simulink model "yoyomodel"  (R2023a)
settings: Solver=VariableStepAuto  StartTime=0.0  StopTime=inf  RelTol=1e-3
values from neighbouring files (symbols this model uses):
  A = [0 ,1; 0, -(e*r)/(I + m*r^2)]    [yoyo.m]
  B = [0; 1/(I + m*r^2)]    [yoyo.m]
  Bi = 1/32.5494    (= 0.0307225325198)    [yoyo.m]
  C = [1 ,0]    [yoyo.m]
  g = 9.81    [yoyo.m]
  K = acker(A,B,[0 0])    [yoyo.m]
  L = acker(A_ccf',C_ccf', [-0.01 -0.01])'    [yoyo.m]
  m = 0.1    [yoyo.m]
  r = 0.035    [yoyo.m]
  x0 = [0; 0]    [yoyo.m]
settings Model: Creator=aditya  LastModifiedBy=aditya
settings SolverCC: ZeroCrossAlgorithm=Adaptive
settings DataIOCC: Refine=5
settings DebuggingCC: IgnoredZcDiagnostic=none

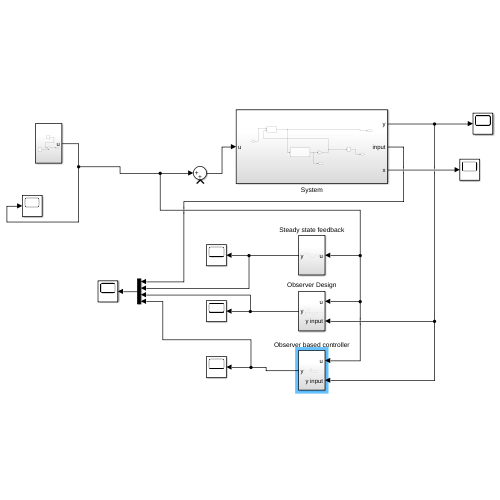
[thumbnail: Simulink's stored preview of the top-level diagram]
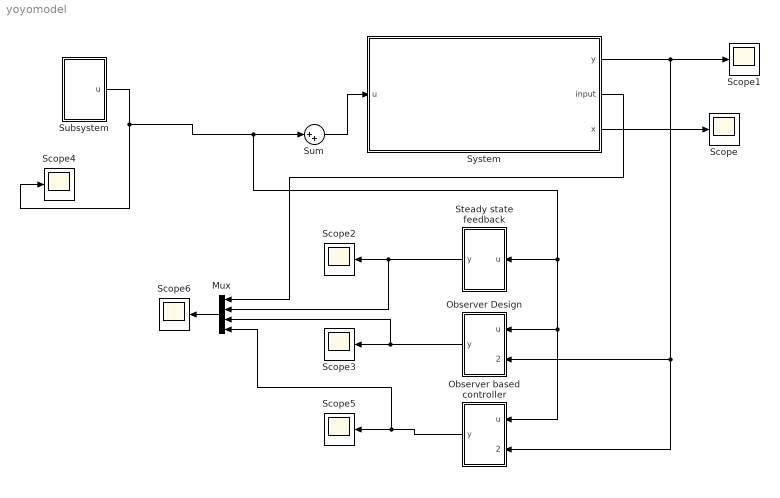
== system yoyomodel ==
  Mux : Mux
  Observer Design : Subsystem
  Observer based controller : Subsystem
  Scope{,1..6} (7 alike) : Scope
  Steady state feedback : Subsystem
  Subsystem : Subsystem
  Sum : Sum  Inputs=|++
  System : Subsystem
  wires:
  Subsystem/1(u) -> Observer based controller/1(u), Observer Design/1(u), Steady state feedback/1(u), Sum/1, Scope4/1
  Sum/1 -> System/1(u)
  System/3(x) -> Scope/1
  System/1(y) -> Observer based controller/2(y input), Observer Design/2(y input), Scope1/1
  Observer based controller/1(y) -> Mux/4, Scope5/1
  Steady state feedback/1(y) -> Mux/2, Scope2/1
  Observer Design/1(y) -> Mux/3, Scope3/1
  Mux/1 -> Scope6/1
  System/2(input) -> Mux/1

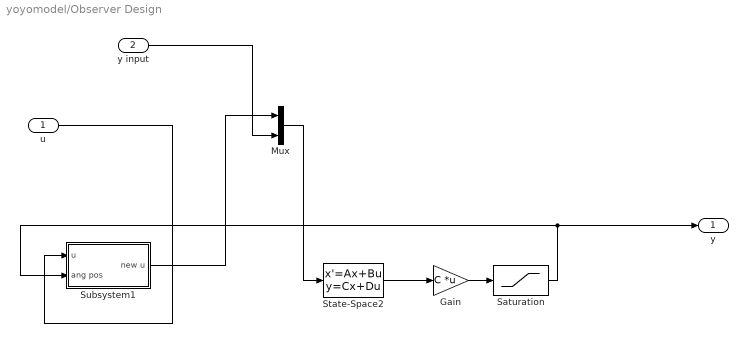
== system yoyomodel/Observer Design ==
  u : Inport
  y input : Inport  Port=2
  Gain : Gain  Gain=C  Multiplication=Matrix(K*u) (u vector)
  Mux : Mux  Inputs=2
  Saturation : Saturate  UpperLimit=123  LowerLimit=0
  State-Space2 : StateSpace  A=A-L*C  B=[B L]  C=eye(2)  D=[0 0;0 0]  InitialCondition=x0
  Subsystem1 : Subsystem
  y : Outport
  wires:
  u/1 -> Subsystem1/1(u)
  State-Space2/1 -> Gain/1
  Saturation/1 -> y/1, Subsystem1/2(ang pos)
  Gain/1 -> Saturation/1
  Mux/1 -> State-Space2/1
  Subsystem1/1(new u) -> Mux/1
  y input/1 -> Mux/2

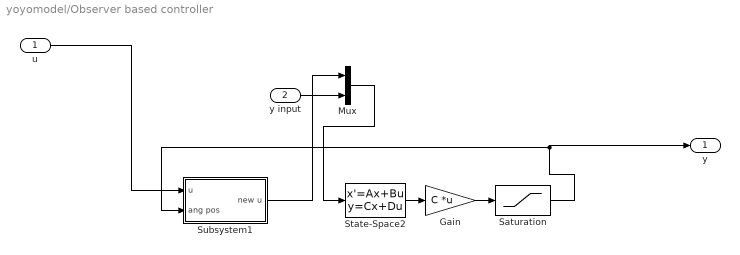
== system yoyomodel/Observer based controller ==
  u : Inport
  y input : Inport  Port=2
  Gain : Gain  Gain=C  Multiplication=Matrix(K*u) (u vector)
  Mux : Mux  Inputs=2
  Saturation : Saturate  UpperLimit=123  LowerLimit=0
  State-Space2 : StateSpace  A=A-B*K-L*C  B=[zeros(size(B)) L]  C=eye(2)  D=[0 0 ;0 0]  InitialCondition=x0
  Subsystem1 : Subsystem
  y : Outport
  wires:
  u/1 -> Subsystem1/1(u)
  State-Space2/1 -> Gain/1
  Saturation/1 -> y/1, Subsystem1/2(ang pos)
  Gain/1 -> Saturation/1
  y input/1 -> Mux/2
  Mux/1 -> State-Space2/1
  Subsystem1/1(new u) -> Mux/1

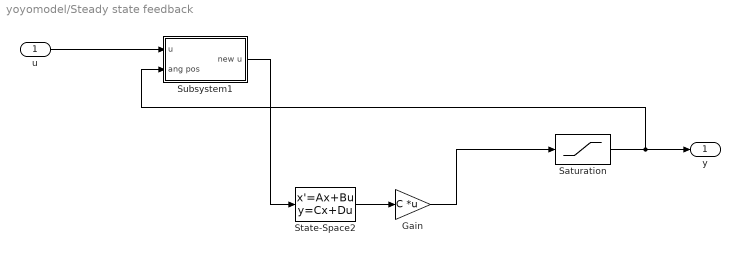
== system yoyomodel/Steady state feedback ==
  u : Inport
  Gain : Gain  Gain=C  Multiplication=Matrix(K*u) (u vector)
  Saturation : Saturate  UpperLimit=123  LowerLimit=0
  State-Space2 : StateSpace  A=A-B*K  B=B  C=eye(2)  D=[0;0]  InitialCondition=x0
  Subsystem1 : Subsystem
  y : Outport
  wires:
  Subsystem1/1(new u) -> State-Space2/1
  u/1 -> Subsystem1/1(u)
  State-Space2/1 -> Gain/1
  Saturation/1 -> Subsystem1/2(ang pos), y/1
  Gain/1 -> Saturation/1

== system yoyomodel/Subsystem ==
  Step1 : Step  Time=0  After=0  SampleTime=0
  Step3 : Step  Time=0  After=0  SampleTime=0
  Sum3 : Sum  Inputs=|+-
  u : Outport
  wires:
  Step3/1 -> Sum3/2
  Step1/1 -> Sum3/1
  Sum3/1 -> u/1

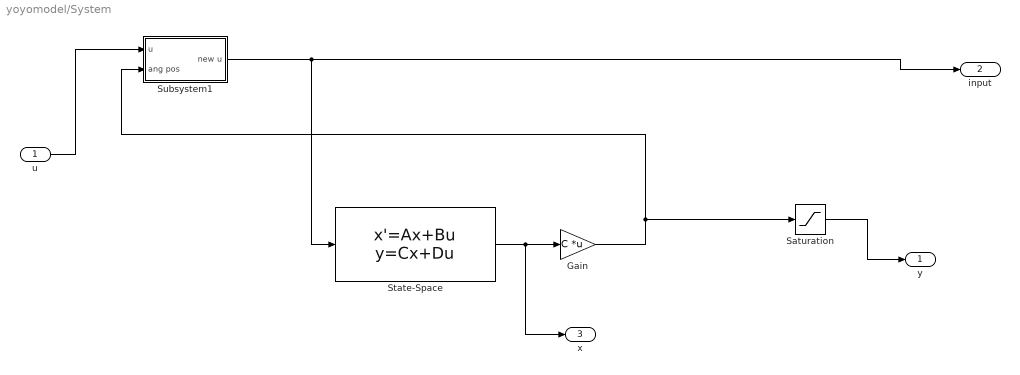
== system yoyomodel/System ==
  u : Inport
  Gain : Gain  Gain=C  Multiplication=Matrix(K*u)
  Saturation : Saturate  UpperLimit=123  LowerLimit=0
  State-Space : StateSpace  A=A  B=B  C=eye(2)  D=[0; 0]  InitialCondition=x0
  Subsystem1 : Subsystem
  y : Outport
  input : Outport  Port=2
  x : Outport  Port=3
  wires:
  Subsystem1/1(new u) -> input/1, State-Space/1
  u/1 -> Subsystem1/1(u)
  State-Space/1 -> x/1, Gain/1
  Saturation/1 -> y/1
  Gain/1 -> Subsystem1/2(ang pos), Saturation/1

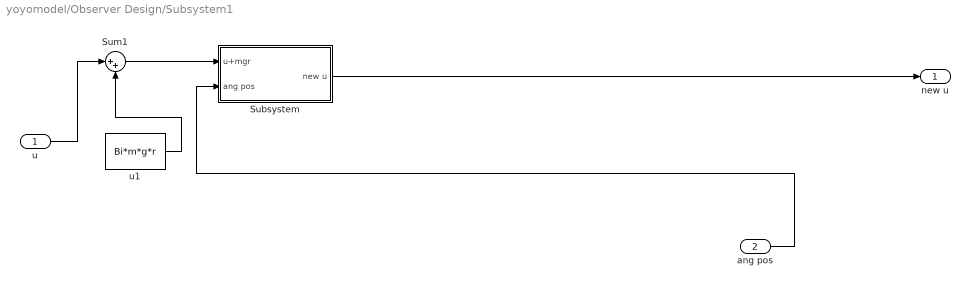
== system yoyomodel/Observer Design/Subsystem1 ==
  u : Inport
  ang pos : Inport  Port=2
  Subsystem : Subsystem
  Sum1 : Sum  Inputs=|++
  u1 : Constant  Value=Bi*m*g*r
  new u : Outport
  wires:
  Sum1/1 -> Subsystem/1(u+mgr)
  u1/1 -> Sum1/2
  ang pos/1 -> Subsystem/2(ang pos)
  Subsystem/1(new u) -> new u/1
  u/1 -> Sum1/1

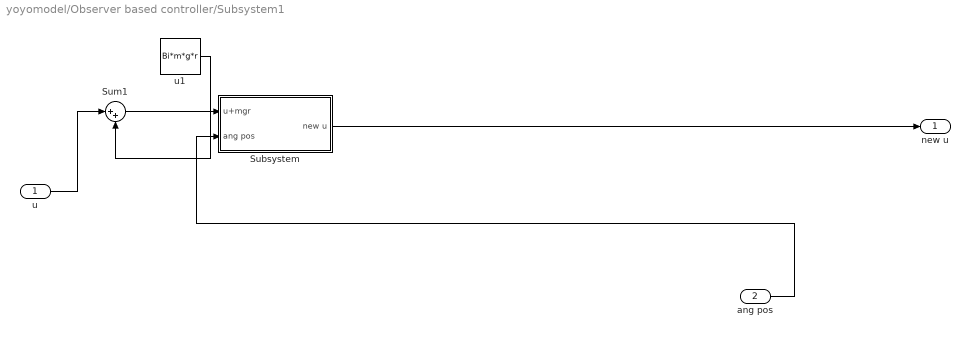
== system yoyomodel/Observer based controller/Subsystem1 ==
  u : Inport
  ang pos : Inport  Port=2
  Subsystem : Subsystem
  Sum1 : Sum  Inputs=|++
  u1 : Constant  Value=Bi*m*g*r
  new u : Outport
  wires:
  Sum1/1 -> Subsystem/1(u+mgr)
  u1/1 -> Sum1/2
  ang pos/1 -> Subsystem/2(ang pos)
  Subsystem/1(new u) -> new u/1
  u/1 -> Sum1/1

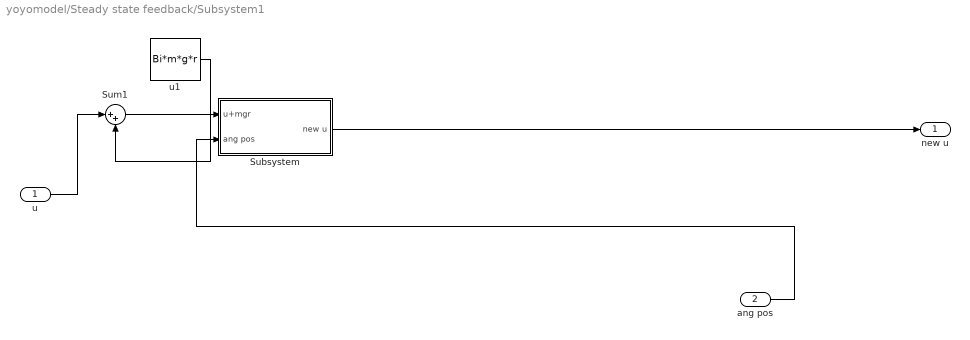
== system yoyomodel/Steady state feedback/Subsystem1 ==
  u : Inport
  ang pos : Inport  Port=2
  Subsystem : Subsystem
  Sum1 : Sum  Inputs=|++
  u1 : Constant  Value=Bi*m*g*r
  new u : Outport
  wires:
  Sum1/1 -> Subsystem/1(u+mgr)
  u1/1 -> Sum1/2
  ang pos/1 -> Subsystem/2(ang pos)
  Subsystem/1(new u) -> new u/1
  u/1 -> Sum1/1

== system yoyomodel/System/Subsystem1 ==
  u : Inport
  ang pos : Inport  Port=2
  Subsystem : Subsystem
  Sum1 : Sum  Inputs=|++
  u1 : Constant  Value=Bi*m*g*r
  new u : Outport
  wires:
  Sum1/1 -> Subsystem/1(u+mgr)
  u1/1 -> Sum1/2
  ang pos/1 -> Subsystem/2(ang pos)
  Subsystem/1(new u) -> new u/1
  u/1 -> Sum1/1

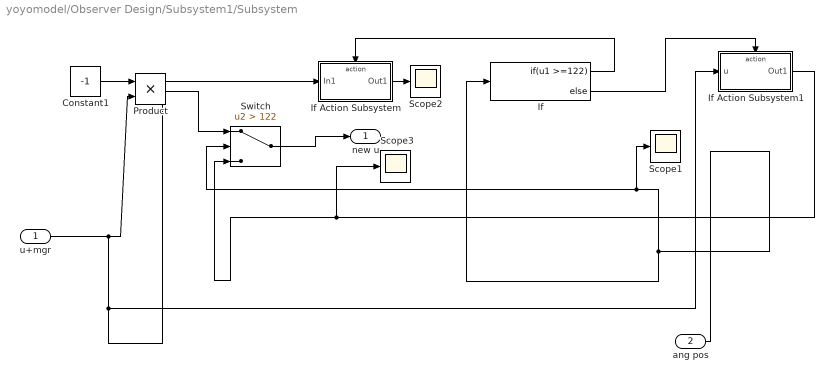
== system yoyomodel/Observer Design/Subsystem1/Subsystem ==
  u+mgr : Inport
  ang pos : Inport  Port=2
  Constant1 : Constant  Value=-1
  If : If  IfExpression=u1 >=122
  If Action Subsystem : Subsystem  TreatAsAtomicUnit=on
  If Action Subsystem1 : Subsystem  TreatAsAtomicUnit=on
  Product : Product
  Scope1 : Scope
  Scope2 : Scope
  Scope3 : Scope
  Switch : Switch  Criteria=u2 > Threshold  Threshold=122  SaturateOnIntegerOverflow=off  InputSameDT=off
  new u : Outport
  wires:
  If Action Subsystem/1(Out1) -> Scope2/1
  If/2 -> If Action Subsystem1/Action
  ang pos/1 -> Scope1/1, Switch/2, If/1
  Product/1 -> Switch/1
  If Action Subsystem1/1(Out1) -> Switch/3, Scope3/1
  Switch/1 -> new u/1
  Constant1/1 -> Product/1
  If/1 -> If Action Subsystem/Action
  u+mgr/1 -> If Action Subsystem/1(In1), If Action Subsystem1/1(u), Product/2

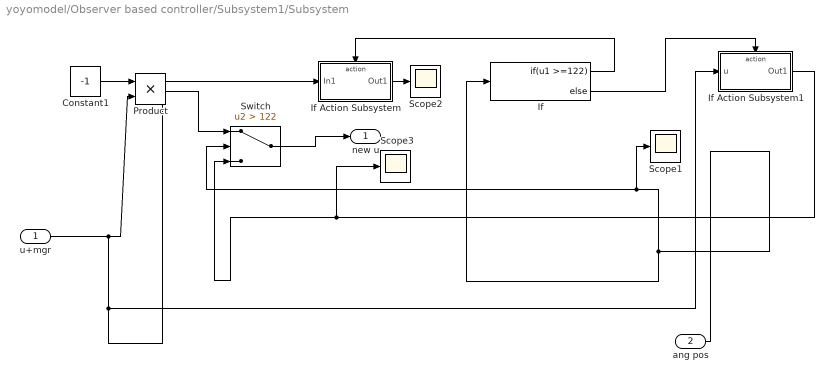
== system yoyomodel/Observer based controller/Subsystem1/Subsystem ==
  u+mgr : Inport
  ang pos : Inport  Port=2
  Constant1 : Constant  Value=-1
  If : If  IfExpression=u1 >=122
  If Action Subsystem : Subsystem  TreatAsAtomicUnit=on
  If Action Subsystem1 : Subsystem  TreatAsAtomicUnit=on
  Product : Product
  Scope1 : Scope
  Scope2 : Scope
  Scope3 : Scope
  Switch : Switch  Criteria=u2 > Threshold  Threshold=122  SaturateOnIntegerOverflow=off  InputSameDT=off
  new u : Outport
  wires:
  If Action Subsystem/1(Out1) -> Scope2/1
  If/2 -> If Action Subsystem1/Action
  ang pos/1 -> Scope1/1, Switch/2, If/1
  Product/1 -> Switch/1
  If Action Subsystem1/1(Out1) -> Switch/3, Scope3/1
  Switch/1 -> new u/1
  Constant1/1 -> Product/1
  If/1 -> If Action Subsystem/Action
  u+mgr/1 -> If Action Subsystem/1(In1), If Action Subsystem1/1(u), Product/2

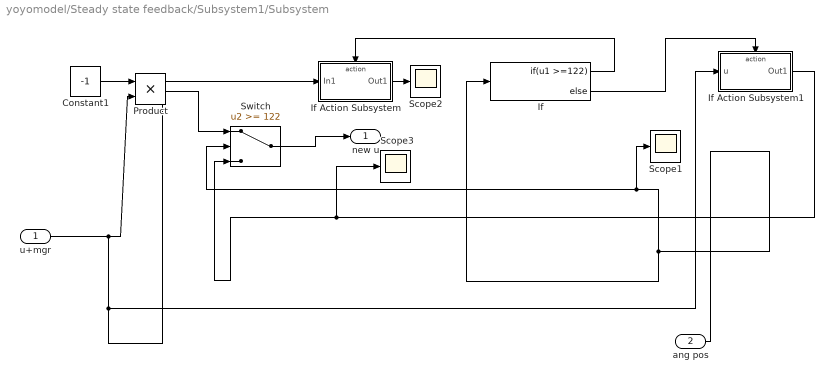
== system yoyomodel/Steady state feedback/Subsystem1/Subsystem ==
  u+mgr : Inport
  ang pos : Inport  Port=2
  Constant1 : Constant  Value=-1
  If : If  IfExpression=u1 >=122
  If Action Subsystem : Subsystem  TreatAsAtomicUnit=on
  If Action Subsystem1 : Subsystem  TreatAsAtomicUnit=on
  Product : Product
  Scope1 : Scope
  Scope2 : Scope
  Scope3 : Scope
  Switch : Switch  Threshold=122  SaturateOnIntegerOverflow=off  InputSameDT=off
  new u : Outport
  wires:
  If Action Subsystem/1(Out1) -> Scope2/1
  If/2 -> If Action Subsystem1/Action
  ang pos/1 -> Scope1/1, Switch/2, If/1
  Product/1 -> Switch/1
  If Action Subsystem1/1(Out1) -> Switch/3, Scope3/1
  Switch/1 -> new u/1
  Constant1/1 -> Product/1
  If/1 -> If Action Subsystem/Action
  u+mgr/1 -> If Action Subsystem/1(In1), If Action Subsystem1/1(u), Product/2

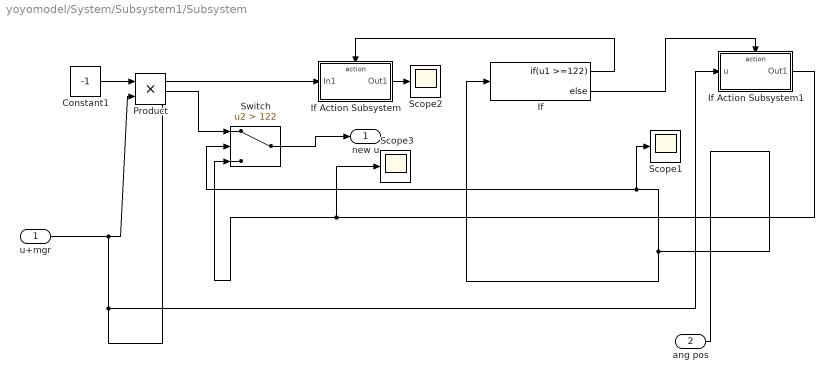
== system yoyomodel/System/Subsystem1/Subsystem ==
  u+mgr : Inport
  ang pos : Inport  Port=2
  Constant1 : Constant  Value=-1
  If : If  IfExpression=u1 >=122
  If Action Subsystem : Subsystem  TreatAsAtomicUnit=on
  If Action Subsystem1 : Subsystem  TreatAsAtomicUnit=on
  Product : Product
  Scope1 : Scope
  Scope2 : Scope
  Scope3 : Scope
  Switch : Switch  Criteria=u2 > Threshold  Threshold=122  SaturateOnIntegerOverflow=off  InputSameDT=off
  new u : Outport
  wires:
  If Action Subsystem/1(Out1) -> Scope2/1
  If/2 -> If Action Subsystem1/Action
  ang pos/1 -> Scope1/1, Switch/2, If/1
  Product/1 -> Switch/1
  If Action Subsystem1/1(Out1) -> Switch/3, Scope3/1
  Switch/1 -> new u/1
  Constant1/1 -> Product/1
  If/1 -> If Action Subsystem/Action
  u+mgr/1 -> If Action Subsystem/1(In1), If Action Subsystem1/1(u), Product/2

== system yoyomodel/Observer Design/Subsystem1/Subsystem/If Action Subsystem ==
  In1 : Inport
  Action Port : ActionPort  ActionPortLabel=if(u1 >=122)
  Out1 : Outport
  wires:
  In1/1 -> Out1/1

== system yoyomodel/Observer Design/Subsystem1/Subsystem/If Action Subsystem1 ==
  u : Inport
  Action Port : ActionPort  ActionPortLabel=else
  Out1 : Outport
  wires:
  u/1 -> Out1/1

== system yoyomodel/Observer based controller/Subsystem1/Subsystem/If Action Subsystem ==
  In1 : Inport
  Action Port : ActionPort  ActionPortLabel=if(u1 >=122)
  Out1 : Outport
  wires:
  In1/1 -> Out1/1

== system yoyomodel/Observer based controller/Subsystem1/Subsystem/If Action Subsystem1 ==
  u : Inport
  Action Port : ActionPort  ActionPortLabel=else
  Out1 : Outport
  wires:
  u/1 -> Out1/1

== system yoyomodel/Steady state feedback/Subsystem1/Subsystem/If Action Subsystem ==
  In1 : Inport
  Action Port : ActionPort  ActionPortLabel=if(u1 >=122)
  Out1 : Outport
  wires:
  In1/1 -> Out1/1

== system yoyomodel/Steady state feedback/Subsystem1/Subsystem/If Action Subsystem1 ==
  u : Inport
  Action Port : ActionPort  ActionPortLabel=else
  Out1 : Outport
  wires:
  u/1 -> Out1/1

== system yoyomodel/System/Subsystem1/Subsystem/If Action Subsystem ==
  In1 : Inport
  Action Port : ActionPort  ActionPortLabel=if(u1 >=122)
  Out1 : Outport
  wires:
  In1/1 -> Out1/1

== system yoyomodel/System/Subsystem1/Subsystem/If Action Subsystem1 ==
  u : Inport
  Action Port : ActionPort  ActionPortLabel=else
  Out1 : Outport
  wires:
  u/1 -> Out1/1
